simulink model "BW2"  (R2016a)
settings: Solver=VariableStepAuto  SolverMode=SingleTasking  StartTime=0.0  StopTime=10.0  RelTol=1e-3
PreLoadFcn:
  | System.m
model workspace: external: MATLAB File C:\Users\darre\Desktop\Measurements\Project simulation Matlab\System.m (data not in the file)
values from neighbouring files (symbols this model uses):
  den1s = [1 (1/(R2*C1)+1/(R1*C1)) 1/(R1*C1*R2*C2)]    [System.m]
  num1s = [1/(R1*C1*R2*C2)]    [System.m]
libraries: simulink_extras x2, simulink x1
settings Model: Creator=darre  LastModifiedBy=darre
settings DataIOCC: LimitDataPoints=on  SaveOutput=off  SaveTime=off
settings OptimizationCC: BlockReduction=off  BooleanDataType=off
settings DebuggingCC: SaveWithParameterizedLinksMsg=none  UnderspecifiedInitializationDetection=Classic  MergeDetectMultiDrivingBlocksExec=none  SignalResolutionControl=TryResolveAllWithWarning  AllowSymbolicDim=off
settings HardwareCC: TargetUnknown=on

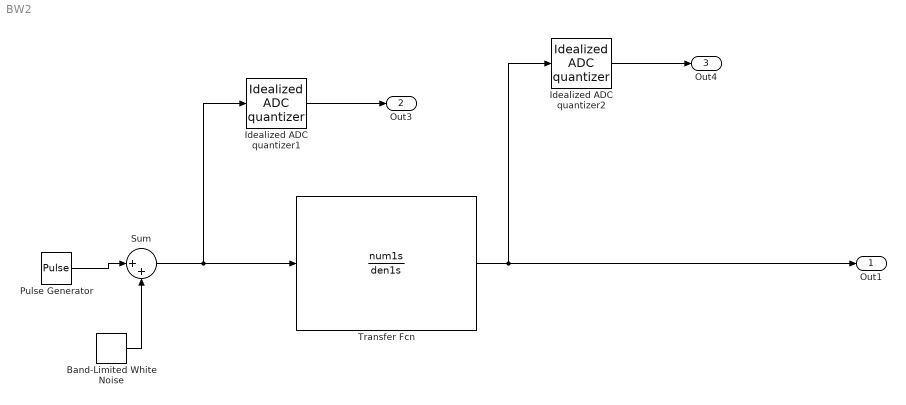
== system BW2 ==
  Band-Limited White Noise : simulink/Sources/Band-Limited White Noise  Cov=[0.000000011]  Ts=0.00001  seed=[230341]
  Idealized ADC quantizer1 : simulink_extras/Additional Discrete/Idealized ADC quantizer  NumberOfConverterBits=12  Vmin=0  Vmax=5.1  OutputDataType=int16  OutputNegativeValues=off
  Idealized ADC quantizer2 : simulink_extras/Additional Discrete/Idealized ADC quantizer  NumberOfConverterBits=12  Vmin=0  Vmax=5.1  OutputDataType=int16  OutputNegativeValues=off
  Pulse Generator : DiscretePulseGenerator  PulseType=Time based  Amplitude=3.3  Period=0.01  PulseWidth=50  PhaseDelay=0.01
  Sum : Sum  Inputs=|++
  Transfer Fcn : TransferFcn  Numerator=num1s  Denominator=den1s
  Out1 : Outport
  Out3 : Outport  Port=2
  Out4 : Outport  Port=3
  wires:
  Transfer Fcn/1 -> Out1/1, Idealized ADC quantizer2/1
  Band-Limited White Noise/1 -> Sum/2
  Pulse Generator/1 -> Sum/1
  Sum/1 -> Idealized ADC quantizer1/1, Transfer Fcn/1
  Idealized ADC quantizer1/1 -> Out3/1
  Idealized ADC quantizer2/1 -> Out4/1
